simulink subsystem "NoSuspensionSSC"  (R2023a)
settings: Solver=VariableStepAuto  StartTime=0.0  StopTime=10.0  RelTol=1e-3
settings Model: Creator=The MathWorks, Inc.  LastModifiedBy=The MathWorks, Inc.

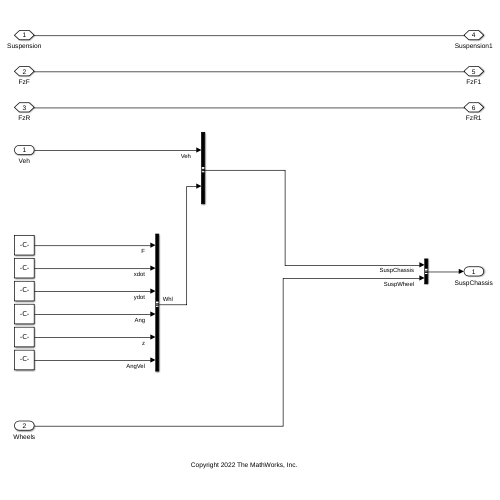
[thumbnail: Simulink's stored preview of the top-level diagram]
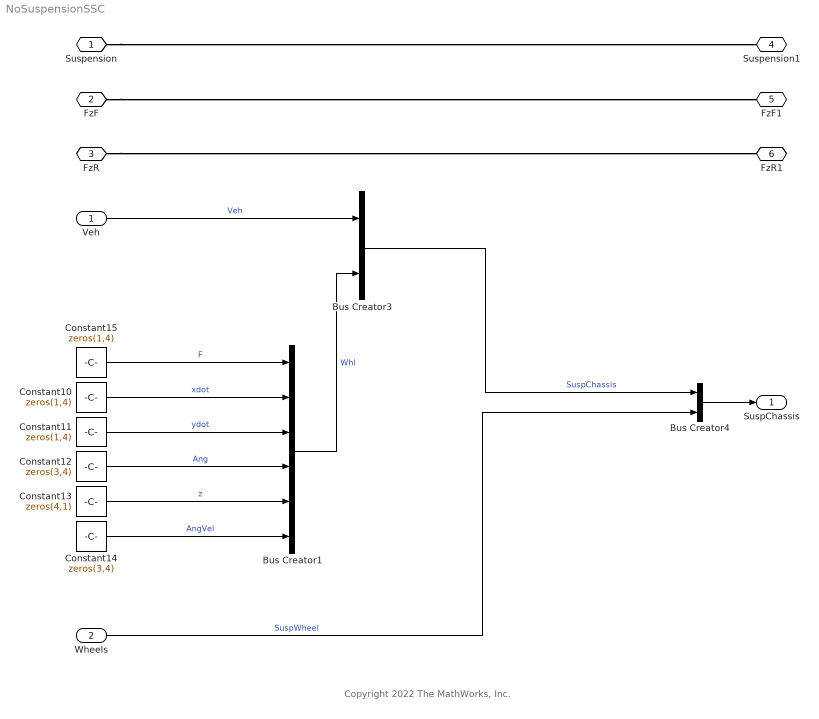
== system NoSuspensionSSC ==
  note: Copyright 2022 The MathWorks, Inc.
  Veh : Inport
  Wheels : Inport  Port=2
  Bus Creator1 : BusCreator  Inputs=6
  Bus Creator3 : BusCreator  Inputs=2
  Bus Creator4 : BusCreator  Inputs=2
  Constant10 : Constant  Value=zeros(1,4)  SampleTime=-1
  Constant11 : Constant  Value=zeros(1,4)  SampleTime=-1
  Constant12 : Constant  Value=zeros(3,4)  SampleTime=-1
  Constant13 : Constant  Value=zeros(4,1)  SampleTime=-1
  Constant14 : Constant  Value=zeros(3,4)  SampleTime=-1
  Constant15 : Constant  Value=zeros(1,4)  SampleTime=-1
  Suspension : PMIOPort  Side=Left
  FzF : PMIOPort  Port=2  Side=Left
  FzR : PMIOPort  Port=3  Side=Left
  Suspension1 : PMIOPort  Port=4  Side=Right
  FzF1 : PMIOPort  Port=5  Side=Right
  FzR1 : PMIOPort  Port=6  Side=Right
  SuspChassis : Outport
  wires:
  Wheels/1 -> Bus Creator4/2  "SuspWheel"
  Constant10/1 -> Bus Creator1/2  "xdot"
  Veh/1 -> Bus Creator3/1  "Veh"
  Bus Creator3/1 -> Bus Creator4/1  "SuspChassis"
  Bus Creator4/1 -> SuspChassis/1
  Bus Creator1/1 -> Bus Creator3/2  "Whl"
  Constant11/1 -> Bus Creator1/3  "ydot"
  Constant12/1 -> Bus Creator1/4  "Ang"
  Constant13/1 -> Bus Creator1/5  "z"
  Constant14/1 -> Bus Creator1/6  "AngVel"
  Constant15/1 -> Bus Creator1/1  "F"
  connections:
  FzR/RConn1 -- FzR1/RConn1
  Suspension/RConn1 -- Suspension1/RConn1
  FzF/RConn1 -- FzF1/RConn1
